simulink model "AltitudeHoldControlS"  (R2018b)
settings: Solver=VariableStepAuto  StartTime=0.0  StopTime=30  RelTol=1e-3
settings Model: Creator=cdjsd  LastModifiedBy=cdjsd

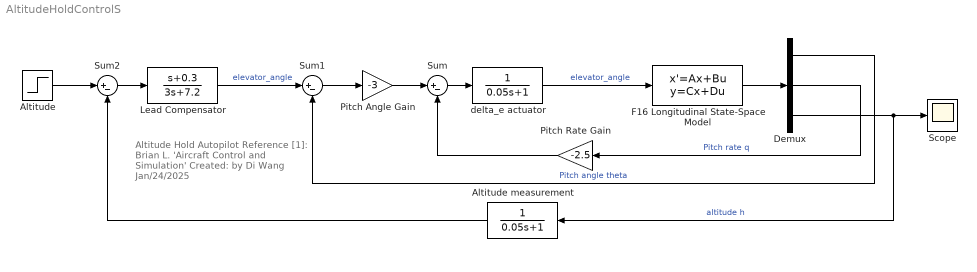
== system AltitudeHoldControlS ==
  note: Altitude Hold Autopilot
      | Reference [1]: Brian L. 'Aircraft Control and Simulation'
      | Created: by Di Wang Jan/24/2025
  Altitude : Step  After=1000  SampleTime=0
  Altitude measurement : TransferFcn  Denominator=[0.05 1]
  Demux : Demux  Outputs=3
  F16 Longitudinal State-Space Model : StateSpace  A=|  B=[0;0;-0.019781;0]  C=|  D=[0;0;0]  InitialCondition=0
      A=|
      | [-0.56761 0 1 2.2633e-6;
      |      0 0 1 0;
      |      -1.4847 0 -0.47599 -1.4947e-7;
      |      -500 500 0 0]
      C=|
      | [0 57.296 0 0;
      |      0 0 57.296 0; 0 0 0 1]
  Lead Compensator : TransferFcn  Numerator=[1 0.3]  Denominator=[3 7.2]
  Pitch Angle Gain : Gain  Gain=-3
  Pitch Rate Gain : Gain  Gain=-2.5
  Scope : Scope
  Sum : Sum  Inputs=|+-
  Sum1 : Sum  Inputs=|+-
  Sum2 : Sum  Inputs=|+-
  delta_e actuator : TransferFcn  Denominator=[0.05 1]
  wires:
  delta_e actuator/1 -> F16 Longitudinal State-Space Model/1  "elevator_angle"
  F16 Longitudinal State-Space Model/1 -> Demux/1
  Demux/3 -> Scope/1, Altitude measurement/1  "altitude h"
  Demux/2 -> Pitch Rate Gain/1  "Pitch rate q"
  Sum/1 -> delta_e actuator/1
  Pitch Rate Gain/1 -> Sum/2
  Pitch Angle Gain/1 -> Sum/1
  Sum1/1 -> Pitch Angle Gain/1
  Demux/1 -> Sum1/2  "Pitch angle theta"
  Lead Compensator/1 -> Sum1/1  "elevator_angle"
  Sum2/1 -> Lead Compensator/1
  Altitude/1 -> Sum2/1
  Altitude measurement/1 -> Sum2/2
